simulink model "singleline_from_pendulum"  (R2020a)
settings: Solver=VariableStepAuto  StartTime=0.0  StopTime=10.0  RelTol=1e-3
undefined symbols (not defined in the file): L, lambda0, m, u0, x0
settings Model: Creator=Pｈｉｌ  LastModifiedBy=Pｈｉｌ

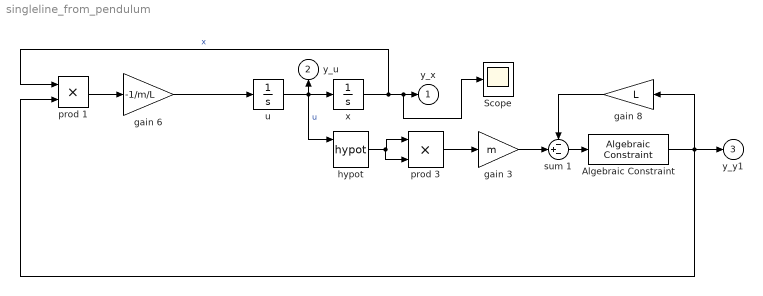
== system singleline_from_pendulum ==
  Algebraic Constraint : AlgebraicConstraint  Solver=Trust region  InitialGuess=-lambda0
  Scope : Scope
  gain 3 : Gain  Gain=m
  gain 6 : Gain  Gain=-1/m/L
  gain 8 : Gain  Gain=L
  hypot : Math  Operator=hypot  SignedPower=on  SaturateOnIntegerOverflow=on
  prod 1 : Product
  prod 3 : Product
  sum 1 : Sum  Inputs=-+-
  u : Integrator  InitialCondition=u0
  x : Integrator  InitialCondition=x0
  y_x : Outport  VectorParamsAs1DForOutWhenUnconnected=off
  y_u : Outport  Port=2  VectorParamsAs1DForOutWhenUnconnected=off
  y_y1 : Outport  Port=3  VectorParamsAs1DForOutWhenUnconnected=off
  wires:
  u/1 -> hypot/1, y_u/1, x/1  "u"
  gain 8/1 -> sum 1/1
  hypot/1 -> prod 3/2, prod 3/1
  gain 3/1 -> sum 1/2
  Algebraic Constraint/1 -> y_y1/1, gain 8/1, prod 1/2
  prod 1/1 -> gain 6/1
  prod 3/1 -> gain 3/1
  gain 6/1 -> u/1
  x/1 -> Scope/1, y_x/1, prod 1/1  "x"
  sum 1/1 -> Algebraic Constraint/1
